simulink model "delay_bram"  (R2012b)
settings: Solver=ode45  StartTime=0.0  StopTime=99  RelTol=1e-3
libraries: xbsIndex_r4 x6
settings Model: Creator=sgowda  LastModifiedBy=sgowda

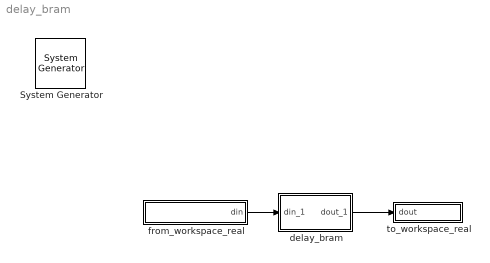
== system delay_bram ==
  " System Generator" : xbsIndex_r4/ System Generator  Tag=genX  xilinxfamily=Kintex7  part=xc7k325t  speed=-3  package=fbg676  synthesis_tool=XST  clock_wrapper=Clock Enables  directory=./netlist  proj_type=Project Navigator  Synth_file=XST Defaults  Impl_file=ISE Defaults  testbench=off  simulink_period=1  sysclk_period=10  dcm_input_clock_period=10  incr_netlist=off  trim_vbits=Everywhere in SubSystem  dbl_ovrd=According to Block Masks  core_generation=According to Block Masks  run_coregen=off  deprecated_control=off  eval_field=0  block_type=sysgen
  delay_bram : Subsystem
  from_workspace_real : Subsystem  mask{var_name=din, n_bits=18, bin_pt=17, quantization=Truncate, overflow=Wrap, arith_type=Signed  (2's comp)}
      mask prompts: var_name "Workspace variable name"; n_bits "# of bits"; bin_pt "Binary Point"; arith_type "Arithmetic type"
      mask init:
      | config.source = str2func('mat_input_data_init_xblock');
      | config.toplevel = gcb();
      | xBlock(config, {config.toplevel, 'var_name', var_name, ...
      |     'n_bits', n_bits, 'bin_pt', bin_pt, 'quantization', quantization, ...
      |     'overflow', overflow, 'arith_type', arith_type});
      mask TypeOptions quantization: Truncate | Round  (unbiased: +/- Inf) | Round  (unbiased: Even Values)
      mask TypeOptions overflow: Wrap | Saturate | Flag as error
      mask TypeOptions arith_type: Signed  (2's comp) | Boolean | Unsigned
  to_workspace_real : Subsystem  mask{var_name=dout}
      mask prompts: var_name "Workspace variable name"
      mask init:
      | config.source = str2func('mat_output_data_init_xblock');
      | config.toplevel = gcb();
      | xBlock(config, {config.toplevel, 'var_name', var_name});
  wires:
  from_workspace_real/1(din) -> delay_bram/1(din_1)
  delay_bram/1(dout_1) -> to_workspace_real/1(dout)

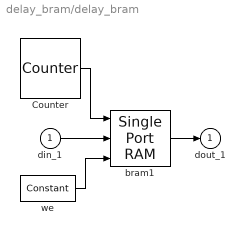
== system delay_bram/delay_bram ==
  din_1 : Inport
  Counter : xbsIndex_r4/Counter  cnt_type=Count Limited  cnt_to=3  operation=Up  start_count=0  cnt_by_val=1  arith_type=Unsigned  n_bits=3  bin_pt=0  load_pin=off  rst=off  en=off  explicit_period=on  period=1  dbl_ovrd=off  use_behavioral_HDL=off  implementation=Fabric  use_rpm=0  block_type=counter
  bram1 : xbsIndex_r4/Single Port RAM  depth=8  initVector=0  distributed_mem=Block RAM  write_mode=Read Before Write  rst=off  init_reg=0  en=off  latency=4  dbl_ovrd=off  optimize=Area  use_rpm=on  block_type=spram
  we : xbsIndex_r4/Constant  const=1  gui_display_data_type=Fixed-point  arith_type=Boolean  n_bits=16  bin_pt=14  preci_type=Single  exp_width=8  frac_width=24  explicit_period=on  period=1  equ=P=C  opselect=C  inp2=PCIN>>17  opr=+  inp1=P  carry=CIN  dbl_ovrd=off  block_type=constant
  dout_1 : Outport
  wires:
  bram1/1 -> dout_1/1
  we/1 -> bram1/3
  din_1/1 -> bram1/2
  Counter/1 -> bram1/1

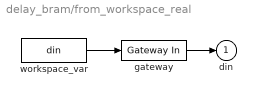
== system delay_bram/from_workspace_real ==
  gateway : xbsIndex_r4/Gateway In  gui_display_data_type=Fixed-point  arith_type="Signed  (2's comp)"  n_bits=18  bin_pt=17  preci_type=Single  exp_width=8  frac_width=24  quantization=Truncate  overflow=Wrap  period=1  dbl_ovrd=off  timing_constraint=None  locs_specified=off  LOCs={}  UseAsADC=off  ADCChannel='1'  inherit_from_input=off  hdl_port=on  block_type=gatewayin
  workspace_var : FromWorkspace  VariableName=din  SampleTime=0
  din : Outport
  wires:
  gateway/1 -> din/1
  workspace_var/1 -> gateway/1

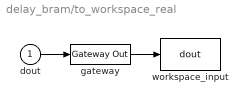
== system delay_bram/to_workspace_real ==
  dout : Inport
  gateway : xbsIndex_r4/Gateway Out  inherit_from_input=on  hdl_port=off  timing_constraint=None  locs_specified=off  LOCs={}  UseAsDAC=off  DACChannel='1'  block_type=gatewayout
  workspace_input : ToWorkspace  VariableName=dout  SampleTime=-1
  wires:
  gateway/1 -> workspace_input/1
  dout/1 -> gateway/1
